simulink model "development_enviroment"  (R2021b)
settings: Solver=VariableStepAuto  StartTime=0.0  StopTime=100  RelTol=1e-3
undefined symbols (not defined in the file or in its folder): A, B, C, D, k1, k3, k_2, tau_1, tau_2, tau_3, zeta
libraries: cstblocks x2
settings Model: Creator=alefr  LastModifiedBy=Alghisi

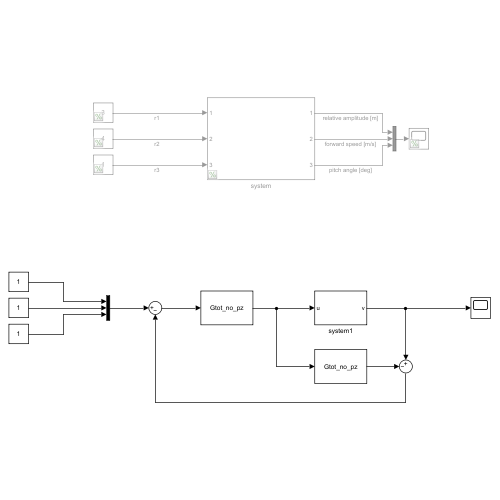
[thumbnail: Simulink's stored preview of the top-level diagram]
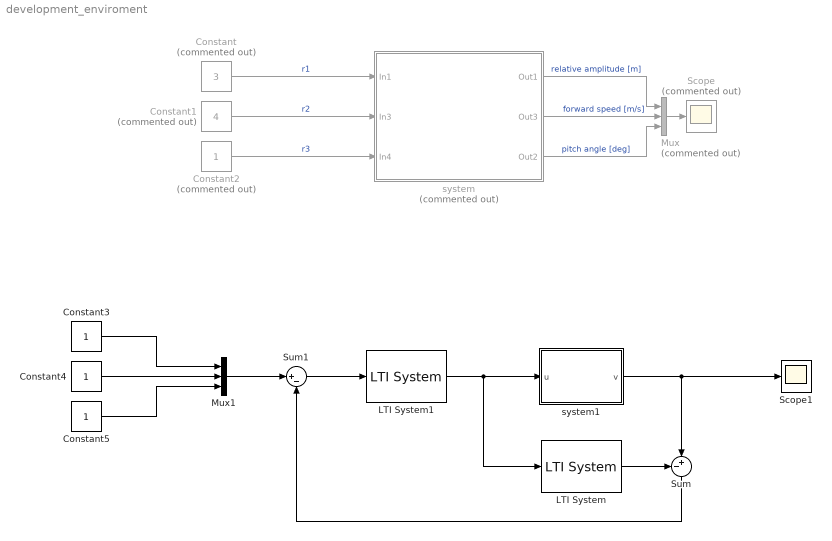
== system development_enviroment ==
  Constant : Constant  Commented=on  Value=3
  Constant1 : Constant  Commented=on  Value=4
  Constant2 : Constant  Commented=on
  Constant3 : Constant
  Constant4 : Constant
  Constant5 : Constant
  LTI System : cstblocks/LTI System  sys=Gtot_no_pz  IC=[]
  LTI System1 : cstblocks/LTI System  sys=Gtot_no_pz  IC=[]
  Mux : Mux  Commented=on  Inputs=3
  Mux1 : Mux  Inputs=3
  Scope : Scope  Commented=on
  Scope1 : Scope
  Sum : Sum  Inputs=-+|
  Sum1 : Sum  Inputs=|+-
  system : Subsystem  Commented=on  mask{k_2_param=mean(k_2), tau_1_param=mean(tau_1), tau_2_param=mean(tau_2), zeta_param=mean(zeta), tau_3_param=mean(tau_3)}
      mask prompts: k_2_param "k_2"; tau_1_param "tau_1"; tau_2_param "tau_2"; zeta_param "zeta"; tau_3_param "tau_3"
  system1 : Subsystem  mask{k_2_param=mean(k_2), tau_1_param=mean(tau_1), tau_2_param=mean(tau_2), zeta_param=mean(zeta), tau_3_param=mean(tau_3)}
      mask prompts: k_2_param "k_2"; tau_1_param "tau_1"; tau_2_param "tau_2"; zeta_param "zeta"; tau_3_param "tau_3"
  wires:
  Constant/1 -> system/1(In1)  "r1"
  Constant1/1 -> system/2(In3)  "r2"
  Constant2/1 -> system/3(In4)  "r3"
  Mux/1 -> Scope/1
  system/1(Out1) -> Mux/1  "relative amplitude [m]"
  system/3(Out2) -> Mux/3  "pitch angle [deg]"
  system/2(Out3) -> Mux/2  "forward speed [m/s]"
  LTI System1/1 -> LTI System/1, system1/1(u)
  system1/1(v) -> Scope1/1, Sum/2
  LTI System/1 -> Sum/1
  Sum1/1 -> LTI System1/1
  Sum/1 -> Sum1/2
  Mux1/1 -> Sum1/1
  Constant3/1 -> Mux1/1
  Constant4/1 -> Mux1/2
  Constant5/1 -> Mux1/3

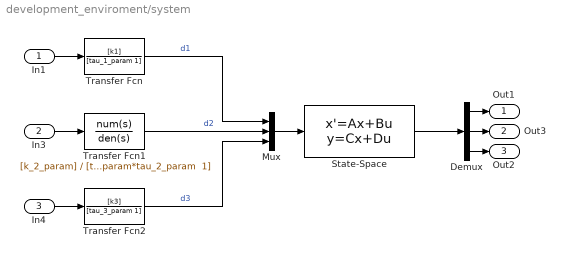
== system development_enviroment/system ==
  In1 : Inport
  In3 : Inport  Port=2
  In4 : Inport  Port=3
  Demux : Demux  Outputs=3
  Mux : Mux  Inputs=3
  State-Space : StateSpace  A=A  B=B  C=C  D=D  InitialCondition=0  ParameterTunability=Unconstrained
      mask Display: image('plane.png'); % Use "Edit Image" on toolstrip to change.
  Transfer Fcn : TransferFcn  Numerator=[k1]  Denominator=[tau_1_param 1]
  Transfer Fcn1 : TransferFcn  Numerator=[k_2_param]  Denominator="[tau_2_param^2  2*zeta_param*tau_2_param  1]"
  Transfer Fcn2 : TransferFcn  Numerator=[k3]  Denominator=[tau_3_param 1]
  Out1 : Outport
  Out3 : Outport  Port=2
  Out2 : Outport  Port=3
  wires:
  State-Space/1 -> Demux/1
  Transfer Fcn/1 -> Mux/1  "d1"
  Transfer Fcn2/1 -> Mux/3  "d3"
  Transfer Fcn1/1 -> Mux/2  "d2"
  Demux/1 -> Out1/1
  Demux/2 -> Out3/1
  Mux/1 -> State-Space/1
  In4/1 -> Transfer Fcn2/1
  In3/1 -> Transfer Fcn1/1
  In1/1 -> Transfer Fcn/1
  Demux/3 -> Out2/1

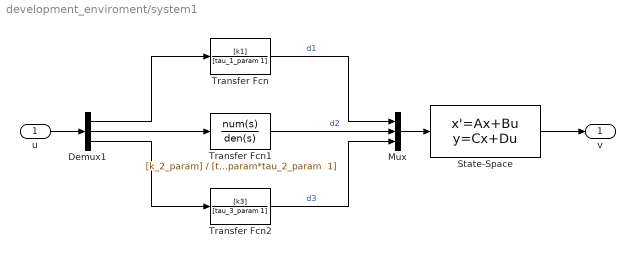
== system development_enviroment/system1 ==
  u : Inport
  Demux1 : Demux  Outputs=3
  Mux : Mux  Inputs=3
  State-Space : StateSpace  A=A  B=B  C=C  D=D  InitialCondition=0  ParameterTunability=Unconstrained
      mask Display: image('plane.png'); % Use "Edit Image" on toolstrip to change.
  Transfer Fcn : TransferFcn  Numerator=[k1]  Denominator=[tau_1_param 1]
  Transfer Fcn1 : TransferFcn  Numerator=[k_2_param]  Denominator="[tau_2_param^2  2*zeta_param*tau_2_param  1]"
  Transfer Fcn2 : TransferFcn  Numerator=[k3]  Denominator=[tau_3_param 1]
  v : Outport
  wires:
  Demux1/1 -> Transfer Fcn/1
  Demux1/2 -> Transfer Fcn1/1
  Demux1/3 -> Transfer Fcn2/1
  Mux/1 -> State-Space/1
  State-Space/1 -> v/1
  Transfer Fcn1/1 -> Mux/2  "d2"
  Transfer Fcn2/1 -> Mux/3  "d3"
  Transfer Fcn/1 -> Mux/1  "d1"
  u/1 -> Demux1/1
